simulink model "thruster_solver"  (R2023a)
settings: Solver=FixedStepAuto  StartTime=0.0  StopTime=inf  FixedStep=.001  RelTol=1e-3
model workspace (MAT data in the model file):
  SL_ROS_VariableLengthArrays_MaxSizes.CommonInfo.ArrayTruncateAction = 'EmitWarning'
  SL_ROS_VariableLengthArrays_MaxSizes.MsgTypeMap = containers.Map
  SL_ROS_VariableLengthArrays_MaxSizes.MsgTypeMap.serialization.keys = {'std_msgs/Float32MultiArray', 'std_msgs/Int16MultiArray', 'std_msgs/Int32MultiArray'}
  SL_ROS_VariableLengthArrays_MaxSizes.MsgTypeMap.serialization.values{1}.PropertyName = 'data'
  SL_ROS_VariableLengthArrays_MaxSizes.MsgTypeMap.serialization.values{1}.DataType = 'single'
  SL_ROS_VariableLengthArrays_MaxSizes.MsgTypeMap.serialization.values{1}.MaxLength = 8
  SL_ROS_VariableLengthArrays_MaxSizes.MsgTypeMap.serialization.values{2}.PropertyName = 'data'
  SL_ROS_VariableLengthArrays_MaxSizes.MsgTypeMap.serialization.values{2}.DataType = 'int16'
  SL_ROS_VariableLengthArrays_MaxSizes.MsgTypeMap.serialization.values{2}.MaxLength = 8
  SL_ROS_VariableLengthArrays_MaxSizes.MsgTypeMap.serialization.values{3}.PropertyName = 'data'
  SL_ROS_VariableLengthArrays_MaxSizes.MsgTypeMap.serialization.values{3}.DataType = 'int32'
  SL_ROS_VariableLengthArrays_MaxSizes.MsgTypeMap.serialization.values{3}.MaxLength = 8
  SL_ROS_VariableLengthArrays_MaxSizes.MsgTypeMap.serialization.uniformity = 0
  SL_ROS_VariableLengthArrays_MaxSizes.MsgTypeMap.serialization.keyType = 'char'
  SL_ROS_VariableLengthArrays_MaxSizes.MsgTypeMap.serialization.valueType = 'any'
undefined symbols (not defined in the file or in its folder): data, data_SL_Info
libraries: ros2lib x19

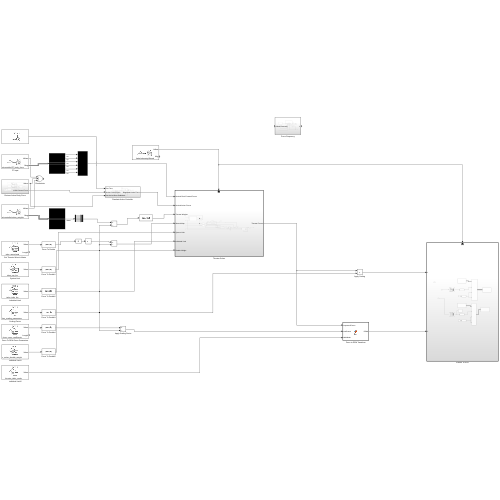
[thumbnail: Simulink's stored preview of the top-level diagram]
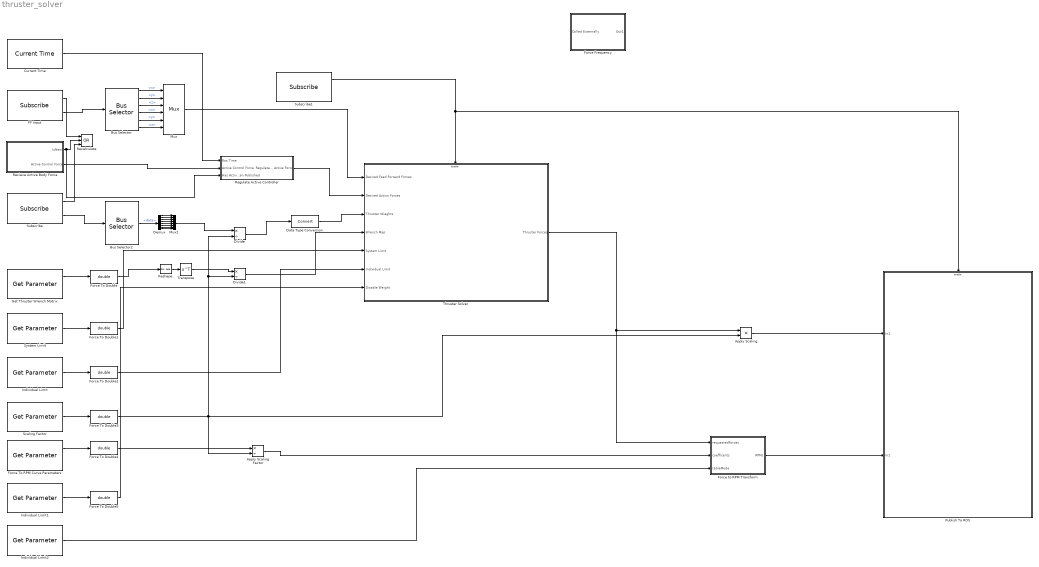
== system thruster_solver ==
  Apply Scaling : Product
  Apply Scaling Factor : Product  Inputs=*/
  Bus Selector : BusSelector  OutputSignals=linear.x,linear.y,linear.z,angular.x,angular.y,angular.z
  Bus Selector2 : BusSelector  OutputSignals=data
  Current Time : ros2lib/Current Time  OutputFormat=double  SampleTime=-1  ModelName=thruster_solver
  Data Type Conversion : DataTypeConversion  SaturateOnIntegerOverflow=off  RndMeth=Floor
  Demux : Demux  Outputs=8
  Divide : Product  Inputs=*/
  Divide1 : Product  Inputs=*/
  FF Input : ros2lib/Subscribe  topicSource=Specify your own  topic=/talos/controller/FF_body_force  messageType=geometry_msgs/Twist  sampleTime=-1  QOSHistory=Keep last  QOSDepth=1  QOSReliability=Reliable  QOSDurability=Volatile
  Force Frequency : Subsystem
  Force To Double{,1..5} (6 alike) : DataTypeConversion  OutDataTypeStr=double  SaturateOnIntegerOverflow=off  RndMeth=Floor
  Force To RPM Curve Parameters : ros2lib/Get Parameter  ParameterName=talos_force_curve_coefficents  ParameterType=int64[]  ParameterMaxArrayLength=8  ParameterInitialValue=[0,0,0,0,0,0,0,0]  SampleTime=-1  ModelName=thruster_solver  BlockId=ParamGet_thruster_solver_205
  Force to RPM Transform : MATLAB Function  TreatAsAtomicUnit=on
  Get Thruster Wrench Matrix : ros2lib/Get Parameter  ParameterName=talos_wrenchmat  ParameterType=int64[]  ParameterMaxArrayLength=48  ParameterInitialValue=0.0  SampleTime=-1  ModelName=thruster_solver  BlockId=ParamGet_thruster_solver_126
  Individual Limit : ros2lib/Get Parameter  ParameterName=talos_indiv_lim  ParameterType=int64  ParameterMaxArrayLength=16  ParameterInitialValue=5.0  SampleTime=-1  ModelName=thruster_solver  BlockId=ParamGet_thruster_solver_147
  Individual Limit1 : ros2lib/Get Parameter  ParameterName=thruster_solver_disable_weight  ParameterType=int64  ParameterMaxArrayLength=16  ParameterInitialValue=10000000  SampleTime=-1  ModelName=thruster_solver  BlockId=ParamGet_thruster_solver_327
  Individual Limit2 : ros2lib/Get Parameter  ParameterName=thruster_table_mode  ParameterType=boolean  ParameterMaxArrayLength=16  ParameterInitialValue=false  SampleTime=-1  ModelName=thruster_solver  BlockId=ParamGet_thruster_solver_335
  Mux : Mux  Inputs=6
  Mux2 : Mux  Inputs=8
  Publish To ROS : Subsystem
  Recalculate : Logic  Operator=OR  Inputs=3  IconShape=distinctive  AllPortsSameDT=off  OutDataTypeStr=boolean
  Recieve Active Body Force : Subsystem
  Regulate Active Controller : Subsystem
  Reshape : Reshape  OutputDimensionality=Customize  OutputDimensions=[6,8]
  Scaling Factor : ros2lib/Get Parameter  ParameterName=thruster_solver_scaling_parameters  ParameterType=int64  ParameterMaxArrayLength=16  ParameterInitialValue=0.0  SampleTime=-1  ModelName=thruster_solver  BlockId=ParamGet_thruster_solver_197
  Subscribe : ros2lib/Subscribe  topicSource=Specify your own  topic=/talos/controller/solver_weights  messageType=std_msgs/Int32MultiArray  sampleTime=-1  QOSHistory=Keep last  QOSDepth=1  QOSReliability=Reliable  QOSDurability=Volatile
  Subscribe1 : ros2lib/Subscribe  topicSource=Specify your own  topic=/talos/odometry/filtered  messageType=nav_msgs/Odometry  sampleTime=0.01  QOSHistory=Keep last  QOSDepth=1  QOSReliability=Reliable  QOSDurability=Volatile
  System Limit : ros2lib/Get Parameter  ParameterName=talos_sys_lim  ParameterType=int64  ParameterMaxArrayLength=16  ParameterInitialValue=10  SampleTime=-1  ModelName=thruster_solver  BlockId=ParamGet_thruster_solver_148
  Thruster Solver : Subsystem
  Transpose : Math  Operator=transpose
  wires:
  FF Input/2 -> Bus Selector/1
  Bus Selector/2 -> Mux/2  "<y>"
  Bus Selector/3 -> Mux/3  "<z>"
  Bus Selector/4 -> Mux/4  "<x>"
  Bus Selector/5 -> Mux/5  "<y>"
  Bus Selector/6 -> Mux/6  "<z>"
  Mux/1 -> Thruster Solver/1(Desired Feed Forward Forces)
  Individual Limit/1 -> Force To Double2/1
  System Limit/1 -> Force To Double1/1
  Get Thruster Wrench Matrix/1 -> Force To Double/1
  Divide1/1 -> Thruster Solver/4(Wrench Map)
  Bus Selector/1 -> Mux/1  "<x>"
  Scaling Factor/1 -> Force To Double3/1
  Reshape/1 -> Transpose/1
  Force To RPM Curve Parameters/1 -> Force To Double4/1
  Apply Scaling Factor/1 -> Force to RPM Transform/2(coefficents)
  Thruster Solver/1(Thruster Forces) -> Force to RPM Transform/1(requestedForces), Apply Scaling/1
  FF Input/1 -> Recalculate/1
  Apply Scaling/1 -> Publish To ROS/1(In1)
  Force to RPM Transform/1(RPMs) -> Publish To ROS/2(In2)
  Transpose/1 -> Divide1/1
  Subscribe/1 -> Recalculate/3
  Divide/1 -> Data Type Conversion/1
  Subscribe/2 -> Bus Selector2/1
  Demux/1 -> Mux2/1
  Demux/2 -> Mux2/2
  Demux/3 -> Mux2/3
  Demux/4 -> Mux2/4
  Demux/5 -> Mux2/5
  Demux/6 -> Mux2/6
  Demux/7 -> Mux2/7
  Demux/8 -> Mux2/8
  Mux2/1 -> Divide/1
  Bus Selector2/1 -> Demux/1  "<data>"
  Data Type Conversion/1 -> Thruster Solver/3(Thruster Wieghts)
  Individual Limit1/1 -> Force To Double5/1
  Individual Limit2/1 -> Force to RPM Transform/3(tableMode)
  Force To Double/1 -> Reshape/1
  Force To Double1/1 -> Thruster Solver/5(System Limit)
  Force To Double2/1 -> Thruster Solver/6(Individual Limit)
  Force To Double3/1 -> Divide/2, Divide1/2, Apply Scaling/2, Apply Scaling Factor/2
  Force To Double4/1 -> Apply Scaling Factor/1
  Force To Double5/1 -> Thruster Solver/7(Disable Weight)
  Recieve Active Body Force/2(Active Control Force) -> Regulate Active Controller/2(Active Control Force)
  Regulate Active Controller/1(Regulated Active Force) -> Thruster Solver/2(Desired Action Forces)
  Recieve Active Body Force/1(IsNew) -> Regulate Active Controller/3(Has Active Been Published), Recalculate/2
  Current Time/1 -> Regulate Active Controller/1(Ros Time)
  Subscribe1/1 -> Publish To ROS/Enable, Thruster Solver/Enable

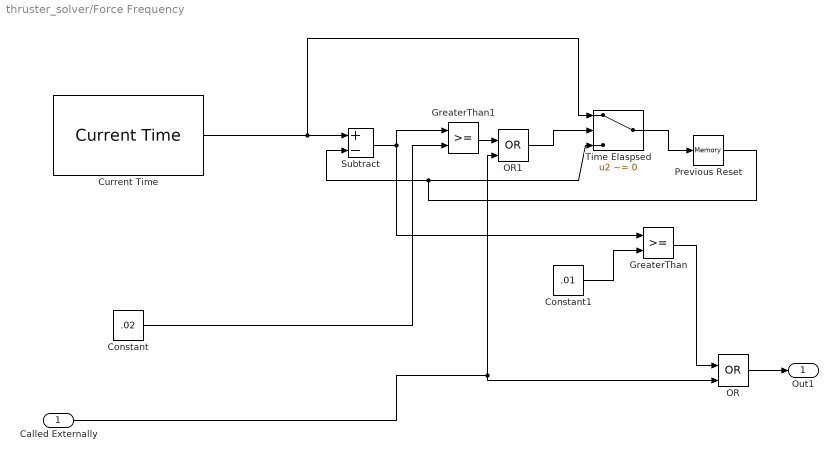
== system thruster_solver/Force Frequency ==
  Called Externally : Inport
  Constant : Constant  Value=.02
  Constant1 : Constant  Value=.01
  Current Time : ros2lib/Current Time  OutputFormat=double  SampleTime=-1  ModelName=thruster_solver
  GreaterThan : RelationalOperator  OutDataTypeStr=boolean  RndMeth=Simplest  InputSameDT=off
  GreaterThan1 : RelationalOperator  OutDataTypeStr=boolean  RndMeth=Simplest  InputSameDT=off
  OR : Logic  Operator=OR  IconShape=distinctive  AllPortsSameDT=off  OutDataTypeStr=boolean
  OR1 : Logic  Operator=OR  IconShape=distinctive  AllPortsSameDT=off  OutDataTypeStr=boolean
  Previous Reset : Memory
  Subtract : Sum  Inputs=+-
  Time Elaspsed : Switch  Criteria=u2 ~= 0  SaturateOnIntegerOverflow=off  InputSameDT=off
  Out1 : Outport
  wires:
  Current Time/1 -> Time Elaspsed/1, Subtract/1
  Time Elaspsed/1 -> Previous Reset/1
  Previous Reset/1 -> Subtract/2, Time Elaspsed/3
  Subtract/1 -> GreaterThan/1, GreaterThan1/1
  GreaterThan/1 -> OR/1
  OR/1 -> Out1/1
  Called Externally/1 -> OR1/2, OR/2
  GreaterThan1/1 -> OR1/1
  OR1/1 -> Time Elaspsed/2
  Constant/1 -> GreaterThan1/2
  Constant1/1 -> GreaterThan/2

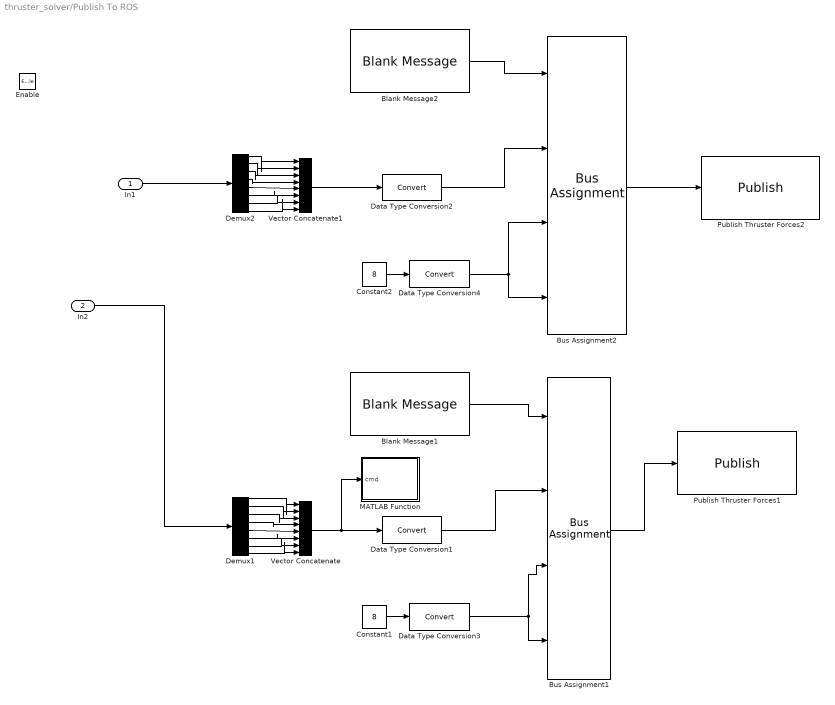
== system thruster_solver/Publish To ROS ==
  In1 : Inport
  In2 : Inport  Port=2
  Enable : EnablePort
  Blank Message1 : ros2lib/Blank Message  messageClass=Message  entityType=std_msgs/Int32MultiArray  messageType=std_msgs/Int32MultiArray  SampleTime=inf
  Blank Message2 : ros2lib/Blank Message  messageClass=Message  entityType=std_msgs/Int32MultiArray  messageType=std_msgs/Int32MultiArray  SampleTime=inf
  Bus Assignment1 : BusAssignment  AssignedSignals=data,data_SL_Info.CurrentLength,data_SL_Info.ReceivedLength
  Bus Assignment2 : BusAssignment  AssignedSignals=data,data_SL_Info.CurrentLength,data_SL_Info.ReceivedLength
  Constant1 : Constant  Value=8
  Constant2 : Constant  Value=8
  Data Type Conversion{1..4} (4 alike) : DataTypeConversion  SaturateOnIntegerOverflow=off  RndMeth=Floor
  Demux1 : Demux  Outputs=8
  Demux2 : Demux  Outputs=8
  MATLAB Function : MATLAB Function  TreatAsAtomicUnit=on
  Publish Thruster Forces1 : ros2lib/Publish  topicSource=Specify your own  topic=/talos/reqRPM  messageType=std_msgs/Int32MultiArray  QOSHistory=Keep last  QOSDepth=1  QOSReliability=Reliable  QOSDurability=Volatile
  Publish Thruster Forces2 : ros2lib/Publish  topicSource=Specify your own  topic=/talos/reqforce  messageType=std_msgs/Int32MultiArray  QOSHistory=Keep last  QOSDepth=1  QOSReliability=Reliable  QOSDurability=Volatile
  Vector Concatenate : Concatenate  NumInputs=8
  Vector Concatenate1 : Concatenate  NumInputs=8
  wires:
  Demux1/8 -> Vector Concatenate/8
  Data Type Conversion2/1 -> Bus Assignment2/2
  Demux1/1 -> Vector Concatenate/1
  Demux2/4 -> Vector Concatenate1/4
  Demux2/5 -> Vector Concatenate1/5
  Demux2/2 -> Vector Concatenate1/2
  Blank Message2/1 -> Bus Assignment2/1
  Demux2/7 -> Vector Concatenate1/7
  Demux1/2 -> Vector Concatenate/2
  Constant2/1 -> Data Type Conversion4/1
  Blank Message1/1 -> Bus Assignment1/1
  Demux2/3 -> Vector Concatenate1/3
  Demux1/6 -> Vector Concatenate/6
  In2/1 -> Demux1/1
  Data Type Conversion4/1 -> Bus Assignment2/3, Bus Assignment2/4
  Vector Concatenate1/1 -> Data Type Conversion2/1
  Demux1/4 -> Vector Concatenate/4
  Bus Assignment2/1 -> Publish Thruster Forces2/1
  Vector Concatenate/1 -> MATLAB Function/1(cmd), Data Type Conversion1/1
  Demux1/5 -> Vector Concatenate/5
  Demux1/3 -> Vector Concatenate/3
  Demux2/8 -> Vector Concatenate1/8
  Demux2/6 -> Vector Concatenate1/6
  Demux1/7 -> Vector Concatenate/7
  Data Type Conversion3/1 -> Bus Assignment1/3, Bus Assignment1/4
  Bus Assignment1/1 -> Publish Thruster Forces1/1
  In1/1 -> Demux2/1
  Data Type Conversion1/1 -> Bus Assignment1/2
  Constant1/1 -> Data Type Conversion3/1
  Demux2/1 -> Vector Concatenate1/1

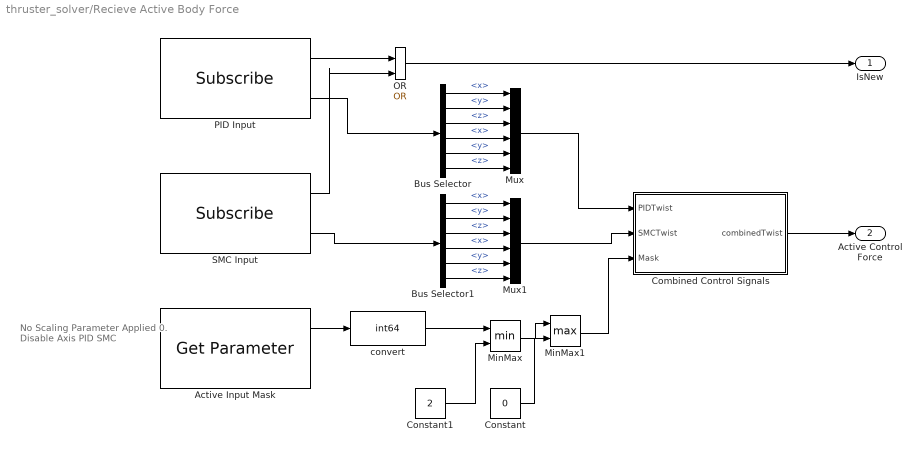
== system thruster_solver/Recieve Active Body Force ==
  note: No Scaling Parameter Applied
      |
      | 0. Disable Axis
      | PID
      | SMC
  Active Input Mask : ros2lib/Get Parameter  ParameterName=active_force_mask  ParameterType=int64[]  ParameterMaxArrayLength=16  ParameterInitialValue=[0,0,0,0,0,0]  SampleTime=-1  ModelName=thruster_solver  BlockId=ParamGet_thruster_solver_394
  Bus Selector : BusSelector  OutputSignals=linear.x,linear.y,linear.z,angular.x,angular.y,angular.z
  Bus Selector1 : BusSelector  OutputSignals=linear.x,linear.y,linear.z,angular.x,angular.y,angular.z
  Combined Control Signals : MATLAB Function  TreatAsAtomicUnit=on
  Constant : Constant  Value=0
  Constant1 : Constant  Value=2
  MinMax : MinMax  Inputs=2
  MinMax1 : MinMax  Function=max  Inputs=2
  Mux : Mux  Inputs=6
  Mux1 : Mux  Inputs=6
  OR : Logic  Operator=OR  IconShape=distinctive  AllPortsSameDT=off  OutDataTypeStr=boolean
  PID Input : ros2lib/Subscribe  topicSource=Specify your own  topic=/talos/controller/active_body_force/pid  messageType=geometry_msgs/Twist  sampleTime=-1  QOSHistory=Keep last  QOSDepth=1  QOSReliability=Reliable  QOSDurability=Volatile
  SMC Input : ros2lib/Subscribe  topicSource=Specify your own  topic=/talos/controller/active_body_force/smc  messageType=geometry_msgs/Twist  sampleTime=-1  QOSHistory=Keep last  QOSDepth=1  QOSReliability=Reliable  QOSDurability=Volatile
  convert : DataTypeConversion  OutMin=0  OutMax=2  OutDataTypeStr=int64  SaturateOnIntegerOverflow=off  RndMeth=Floor
  IsNew : Outport
  Active Control Force : Outport  Port=2
  wires:
  PID Input/1 -> OR/1
  SMC Input/1 -> OR/2
  OR/1 -> IsNew/1
  Combined Control Signals/1(combinedTwist) -> Active Control Force/1
  PID Input/2 -> Bus Selector/1
  Bus Selector/1 -> Mux/1  "<x>"
  Bus Selector/2 -> Mux/2  "<y>"
  Bus Selector/3 -> Mux/3  "<z>"
  Bus Selector/4 -> Mux/4  "<x>"
  Bus Selector/5 -> Mux/5  "<y>"
  Bus Selector/6 -> Mux/6  "<z>"
  Mux/1 -> Combined Control Signals/1(PIDTwist)
  Bus Selector1/6 -> Mux1/6  "<z>"
  Bus Selector1/2 -> Mux1/2  "<y>"
  Bus Selector1/4 -> Mux1/4  "<x>"
  SMC Input/2 -> Bus Selector1/1
  Bus Selector1/5 -> Mux1/5  "<y>"
  Bus Selector1/3 -> Mux1/3  "<z>"
  Bus Selector1/1 -> Mux1/1  "<x>"
  Mux1/1 -> Combined Control Signals/2(SMCTwist)
  Active Input Mask/1 -> convert/1
  convert/1 -> MinMax/1
  MinMax/1 -> MinMax1/1
  MinMax1/1 -> Combined Control Signals/3(Mask)
  Constant/1 -> MinMax1/2
  Constant1/1 -> MinMax/2

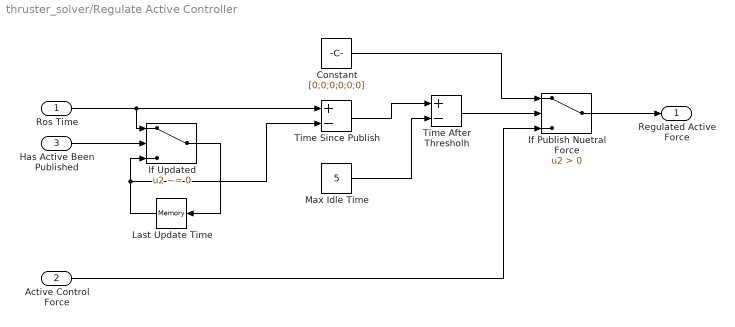
== system thruster_solver/Regulate Active Controller ==
  Ros Time : Inport
  Active Control Force : Inport  Port=2
  Has Active Been Published : Inport  Port=3
  Constant : Constant  Value=[0;0;0;0;0;0]
  If Publish Nuetral Force : Switch  Criteria=u2 > Threshold  SaturateOnIntegerOverflow=off  InputSameDT=off
  If Updated : Switch  Criteria=u2 ~= 0  SaturateOnIntegerOverflow=off  InputSameDT=off
  Last Update Time : Memory
  Max Idle Time : Constant  Value=5
  Time After Thresholh : Sum  Inputs=+-
  Time Since Publish : Sum  Inputs=+-
  Regulated Active Force : Outport
  wires:
  Time After Thresholh/1 -> If Publish Nuetral Force/2
  Max Idle Time/1 -> Time After Thresholh/2
  If Publish Nuetral Force/1 -> Regulated Active Force/1
  Time Since Publish/1 -> Time After Thresholh/1
  Active Control Force/1 -> If Publish Nuetral Force/3
  If Updated/1 -> Last Update Time/1
  Constant/1 -> If Publish Nuetral Force/1
  Has Active Been Published/1 -> If Updated/2
  Last Update Time/1 -> Time Since Publish/2, If Updated/3
  Ros Time/1 -> If Updated/1, Time Since Publish/1

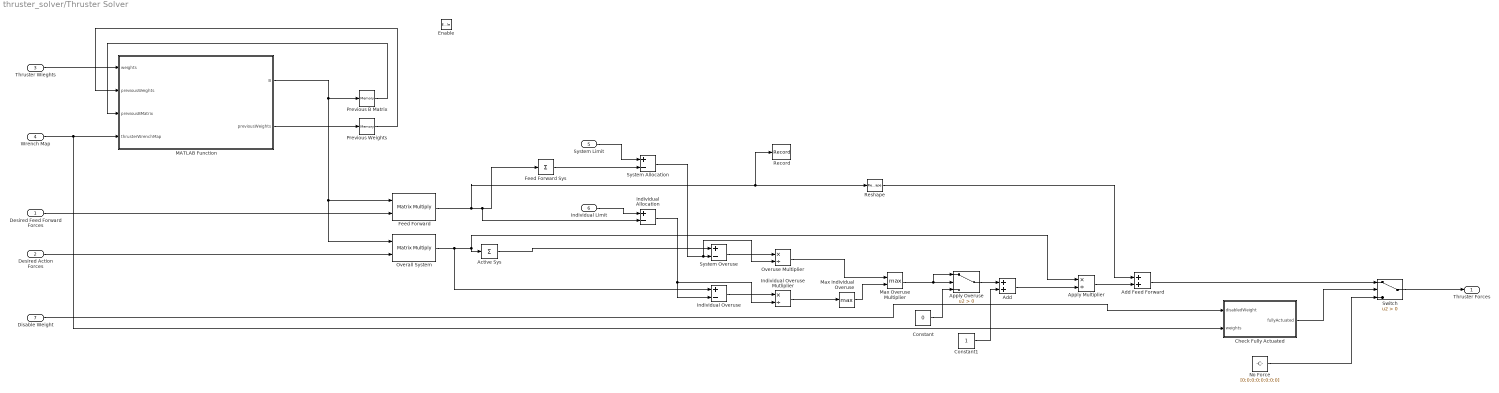
== system thruster_solver/Thruster Solver ==
  Desired Feed Forward Forces : Inport  PortDimensions=[6 1]
  Desired Action Forces : Inport  Port=2  PortDimensions=[6 1]
  Thruster Wieghts : Inport  Port=3  PortDimensions=[8 1]
  Wrench Map : Inport  Port=4
  System Limit : Inport  Port=5
  Individual Limit : Inport  Port=6
  Disable Weight : Inport  Port=7
  Enable : EnablePort
  Active Sys : Sum  Inputs=+
  Add : Sum
  Add Feed Forward : Sum  AccumDataTypeStr=double
  Apply Multiplier : Product  Inputs=*/  OutDataTypeStr=double
  Apply Overuse : Switch  Criteria=u2 > Threshold  SaturateOnIntegerOverflow=off  InputSameDT=off
  Check Fully Actuated : MATLAB Function  TreatAsAtomicUnit=on
  Constant : Constant  Value=0
  Constant1 : Constant
  "Feed Forward " : Product  Multiplication=Matrix(*)
  Feed Forward Sys : Sum  Inputs=+
  Individual Allocation : Sum  Inputs=+-
  Individual Overuse : Sum  Inputs=+-
  Individual Overuse Mutliplier : Product  Inputs=*/
  MATLAB Function : MATLAB Function  TreatAsAtomicUnit=on
  Max Individual Overuse : MinMax  Function=max
  Max Overuse Multiplier : MinMax  Function=max  Inputs=2
  No Force : Constant  Value=[0;0;0;0;0;0;0;0]
  Overall System : Product  Multiplication=Matrix(*)
  Overuse Multiplier : Product  Inputs=*/
  Previous B Matrix : Memory  InitialCondition=[inf inf inf inf inf inf; inf inf inf inf inf inf; inf inf inf inf inf inf; inf inf inf inf inf inf; inf inf inf inf inf inf; inf inf inf inf inf inf; inf inf inf inf inf inf; inf inf inf inf inf inf]  InheritSampleTime=on
  Previous Weights : Memory  InitialCondition=[ inf inf inf inf inf inf inf inf]  InheritSampleTime=on
  Record : Record  FileSettingsInternal="{\"entries\":[{\"content\":{\"excelSettings\":{\"content\":{},\"type\":\"Streamout.ExcelSettings\"}},\"type\":\"Streamout.FileSettingStorage\",\"uuid\":\"\"}],\"packageUris\":[\"http:\\/\\/schema.mathworks.com\\/mf0\\/streamout_blocks\\/R2020a\"],\"version\":\"1.0\"}"  SignalsInternal="{\"entries\":[{\"content\":{\"signals\":[{\"content\":{\"blockPath\":[],\"dimensions\":[8,1],\"domain\":\"\",\"hasChildren\":true,\"lineColor\":\"#edb120\",\"port\":1,\"sid\":[\"\"],\"signalID\":2007,\"signalName\":\"Feed Forward \"},\"type\":\"RecordBlkView.Signal\",\"uuid\":\"\"},{\"content\":{\"blockPath\":[],\"channel\":[1,1],\"dimensions\":[8,1],\"domain\":\"\",\"lineColor\":\"#d95319\",\"parentID\":2007,\"plots\":[1],\"port\":1,\"sid\":[\"\"],\"signalID\":2008 ...(+1786 chars)"  VisualizationBindings="{\"sparklinesplugin\":{\"info\":[{\"bindingParametersList\":[],\"subplotID\":1}]}}"
  Reshape : Reshape  OutputDimensionality=Column vector (2-D)
  Switch : Switch  Criteria=u2 > Threshold  SaturateOnIntegerOverflow=off  InputSameDT=off
  System Allocation : Sum  Inputs=+-
  System Overuse : Sum  Inputs=+-
  Thruster Forces : Outport
  wires:
  Constant/1 -> Apply Overuse/3
  Feed Forward Sys/1 -> System Allocation/2
  Individual Overuse/1 -> Individual Overuse Mutliplier/1
  Individual Allocation/1 -> Individual Overuse Mutliplier/2, Individual Overuse/2
  Overall System/1 -> Individual Overuse/1, Apply Multiplier/1, Active Sys/1
  Max Overuse Multiplier/1 -> Apply Overuse/1, Apply Overuse/2
  Desired Feed Forward Forces/1 -> "Feed Forward "/2
  System Overuse/1 -> Overuse Multiplier/1
  Active Sys/1 -> System Overuse/1
  Apply Multiplier/1 -> Add Feed Forward/2
  Overuse Multiplier/1 -> Max Overuse Multiplier/1
  Max Individual Overuse/1 -> Max Overuse Multiplier/2
  System Allocation/1 -> Overuse Multiplier/2, System Overuse/2
  Desired Action Forces/1 -> Overall System/2
  "Feed Forward "/1 -> Record/1, Reshape/1, Individual Allocation/2, Feed Forward Sys/1
  Constant1/1 -> Add/2
  Individual Overuse Mutliplier/1 -> Max Individual Overuse/1
  Apply Overuse/1 -> Add/1
  Add/1 -> Apply Multiplier/2
  Add Feed Forward/1 -> Switch/1
  MATLAB Function/1(B) -> Overall System/1, "Feed Forward "/1, Previous B Matrix/1
  Previous B Matrix/1 -> MATLAB Function/3(previousBMatrix)
  Wrench Map/1 -> Check Fully Actuated/2(weights), MATLAB Function/4(thrusterWrenchMap)
  Thruster Wieghts/1 -> MATLAB Function/1(weights)
  Previous Weights/1 -> MATLAB Function/2("previousWeights ")
  System Limit/1 -> System Allocation/1
  Individual Limit/1 -> Individual Allocation/1
  MATLAB Function/2(previousWeights) -> Previous Weights/1
  Reshape/1 -> Add Feed Forward/1
  Check Fully Actuated/1(fullyActuated) -> Switch/2
  Disable Weight/1 -> Check Fully Actuated/1(disabledWeight)
  No Force/1 -> Switch/3
  Switch/1 -> Thruster Forces/1

== matlab function thruster_solver/Force to RPM Transform ==
function RPMs = fcn(requestedForces, coefficents, tableMode)

%the output array with rpm values
RPMs = zeros([8,1]);

if(tableMode)
   %evaluate each thruster -- discontinuos curve
    for i = 1:8
        requestedForce = requestedForces(i);
    
        if(requestedForce > .01)
            %positive curve
            RPMs(i) = 120 + sin(requestedForce/ 60 * pi) ^ (1/3) * 130;
            RPMs(i) = min(250, RPMs(i));
        elseif(requestedForce < -.01)
            %negative curve
            RPMs(i) = -120 - (abs(sin(requestedForce/ 60 * pi)) ^ (1/3)) * 130;
            RPMs(i) = max(-250, RPMs(i));  
        end
    end 

else

    %evaluate each thruster -- discontinuos curve
    for i = 1:8
        requestedForce = requestedForces(i);
        
        if(requestedForce > 0)
            %positive curve
            RPMs(i) = round(coefficents(1) + coefficents(2) * requestedForces(i) + coefficents(3) * tanh(requestedForces(i)) + requestedForces(i)^(1/4) * coefficents(4));
        else
            %negative curve
            RPMs(i) = round(coefficents(5) + coefficents(6) * requestedForces(i) + coefficents(7) * tanh(requestedForces(i)) + abs(requestedForces(i))^(1/4) * coefficents(8));
        end
    
    end

end

== matlab function thruster_solver/Thruster Solver/MATLAB Function ==
function [B,previousWeights] = generateBMatrix(weights, previousWeights, previousBMatrix, thrusterWrenchMap)

    if(isequal(weights, previousWeights))
        %if the weights are the same, just send the previous B matrix
        B = previousBMatrix;
        return
    end

    %if new weights, calculate the a new b matrix
    weightsMatrix = diag(weights);
    B = inv(weightsMatrix) * (thrusterWrenchMap) * inv((transpose(thrusterWrenchMap) * inv(weightsMatrix) * (thrusterWrenchMap)))
    previousWeights = weights;
end

== matlab function thruster_solver/Thruster Solver/Check Fully Actuated ==
function fullyActuated = fcn(disabledWeight, weights)

enabled_thrusters = 0;

%count number of enabled thrusters
for i = 1:length(weights)
    if(weights(i) < disabledWeight)
        enabled_thrusters = enabled_thrusters + 1;
    end
end

%if enough thrusters to be fully actuated allow forces
if(enabled_thrusters >= 6)
    fullyActuated = 1;

    return
end

fullyActuated = 0;

== matlab function thruster_solver/Recieve Active Body Force/Combined Control Signals ==
function combinedTwist = fcn(PIDTwist, SMCTwist, Mask)

combinedTwist = zeros(6,1);

controlArray = [[0;0;0;0;0;0],  PIDTwist, SMCTwist];

%get control value from array
for i=1:6
    combinedTwist(i) = controlArray(i, Mask(i) + 1);
end

== matlab function thruster_solver/Publish To ROS/MATLAB Function ==
function fcn(cmd)
send_thruster_cmd(cmd);
